simulink model "Simulink_MPC"  (R2022a)
settings: Solver=FixedStepAuto  StartTime=0.0  StopTime=2000  FixedStep=1e-2  RelTol=1e-3
values from neighbouring files (symbols this model uses):
  A = [-b/J K/J ... (first row only)    [Generic_MPC.m]    (also in Koopman.m = zeros(nx,size(X,1)))
  B = [0 ... (first row only)    [Generic_MPC.m]    (also in Koopman.m = zeros(nx,size(U,1)))
  C = eye(2)    [Generic_MPC.m]    (also in Koopman_Eigen.m = Unobserver(Py,Z); Koopman_Lifting.m = Unobserver(Py,Z))
  D = zeros(2,1)    [Generic_MPC.m]    (also in Koopman_Eigen.m = zeros(size(Z,1),size(U,1)); Koopman_Lifting.m = zeros(size(Z,1),size(U,1)))
libraries: mpclib x1
settings Model: Creator=sergiovaneg  LastModifiedBy=sergiovaneg
settings DataIOCC: SaveOutput=off  DSMLogging=off  ReturnWorkspaceOutputs=off

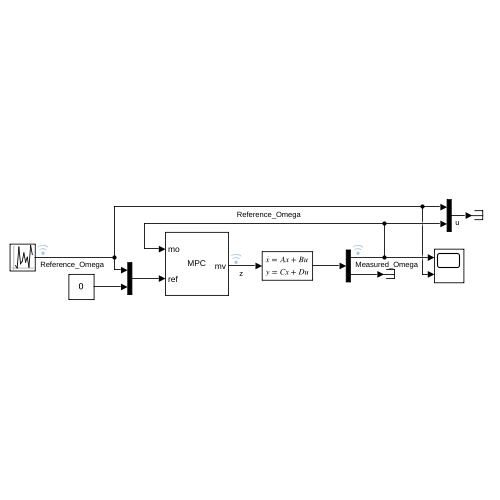
[thumbnail: Simulink's stored preview of the top-level diagram]
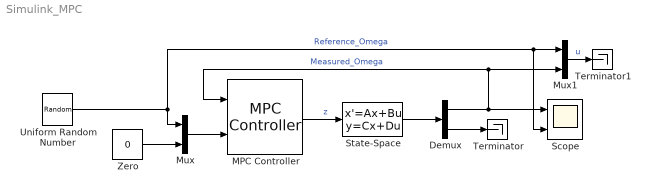
== system Simulink_MPC ==
  Demux : Demux  Outputs=2
  MPC Controller : mpclib/MPC Controller  SCDEnableBlockLinearizationSpecification=on  mpcobj=DC_Motor_MPC  is_multiple=0  enable_value=0  return_u0=off  updateMPCinCallerWorkspace=on  md_inport=off  mv_inport=off  uref_inport=off  return_cost=off  return_mvseq=off  return_qpstatus=off  return_xseq=off  return_state=off  return_ovseq=off  state_inport=off  umin_inport=off  umax_inport=off  ymin_inport=off  ymax_inport=off  cc_inport=off  ywt_inport=off  uwt_inport=off  duwt_inport=off  rhoeps_inport=off  pm_inport=off  MaximumP=10  HorizonChoice=FixedHorizon  n_ts=0.01  n_p=10  n_mv=1  n_md=0  n_ud=0  n_mo=1  n_uo=1  BlockDataType=double  SampleTimeInherited=off  switch_inport=off
  Mux : Mux  Inputs=2
  Mux1 : Mux  Inputs=2
  Scope : Scope  NumInputPorts=2
  State-Space : StateSpace  A=A  B=B  C=C  D=D  InitialCondition=0
  Terminator : Terminator
  Terminator1 : Terminator
  Uniform Random Number : UniformRandomNumber  SampleTime=0.01
  Zero : Constant  Value=0  OutDataTypeStr=Inherit: Inherit via back propagation
  wires:
  MPC Controller/1 -> State-Space/1  "z"
  State-Space/1 -> Demux/1
  Demux/1 -> Scope/1, Mux1/2, MPC Controller/1  "Measured_Omega"
  Mux/1 -> MPC Controller/2
  Uniform Random Number/1 -> Mux/1, Scope/2, Mux1/1  "Reference_Omega"
  Zero/1 -> Mux/2
  Demux/2 -> Terminator/1
  Mux1/1 -> Terminator1/1  "u"
